simulink model "bmw_roadster"  (R2022b)
settings: Solver=ode45  StartTime=0.0  StopTime=15  RelTol=1e-3  EnableMultiTasking=on
PreLoadFcn:
  | % Parameters
  | load gear_data;
  | FDR = 3.23;
  | AvgEngTorque = 222;
  | Loss = 0.8;
  | r_tire = 1.030;
  | m = 104.2;
  | Cd = 0.4;
  | rho = 2.377e-3;
  | h = 4.15;
  | w = 5.71;
settings Model: Creator=jrivitus  LastModifiedBy=bensweet
settings SolverCC: AlgebraicLoopSolver=TrustRegion
settings DataIOCC: ExternalInput=[t, gear]  LimitDataPoints=on  LoadExternalInput=on  SaveFormat=Array  ReturnWorkspaceOutputs=off
settings OptimizationCC: ExpressionDepthLimit=2147483647  LifeSpan=inf
settings DebuggingCC: UnconnectedInputMsg=warning  UnconnectedOutputMsg=warning  UnconnectedLineMsg=warning  PregeneratedLibrarySubsystemCodeDiagnostic=none  SFMachineParentedDataDiag=warning
settings HardwareCC: ProdBitPerPointer=32  ProdBitPerSizeT=32  ProdBitPerPtrDiffT=32  ProdLargestAtomicFloat=None  ProdIntDivRoundTo=Undefined  ProdEndianess=Unspecified  ProdWordSize=32  ProdHWDeviceType=32-bit Generic
settings ModelReferenceCC: EnableRefExpFcnMdlSchedulingChecks=on  PropagateSignalLabelsOutOfModel=off
settings SFSimCC: SimUseLocalCustomCode=off
settings RTWCC: RTWUseLocalCustomCode=off  DLArmComputeVersion=19.05
settings CodeAppCC: StateflowObjectComments=on
settings GRTTargetCC: TargetLangStandard=C89/C90 (ANSI)  CombineOutputUpdateFcns=off  GRTInterface=on
settings ConfigComp: CovMetricSettings=dw  CovSaveCumulativeToWorkspaceVar=on  CovSaveSingleToWorkspaceVar=on  CovExternalEMLEnable=off  CovSFcnEnable=off

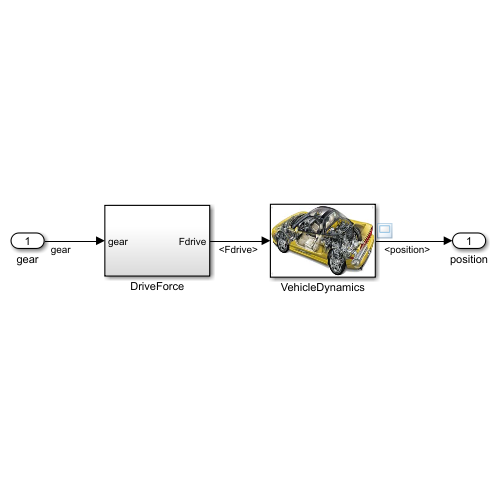
[thumbnail: Simulink's stored preview of the top-level diagram]
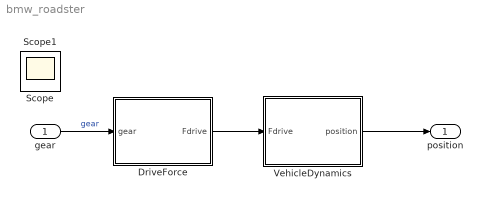
== system bmw_roadster ==
  gear : Inport
  DriveForce : Subsystem
  VehicleDynamics : Subsystem
      mask Display: image("carImg.jpg")
  position : Outport  VectorParamsAs1DForOutWhenUnconnected=off
  Scope : Scope
  Scope1 : Scope
  wires:
  DriveForce/1(Fdrive) -> VehicleDynamics/1(Fdrive)
  gear/1 -> DriveForce/1(gear)  "gear"
  VehicleDynamics/1(position) -> position/1

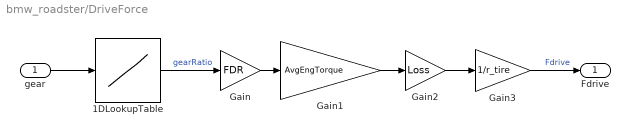
== system bmw_roadster/DriveForce ==
  gear : Inport
  1DLookupTable : Lookup_n-D  NumberOfTableDimensions=1  BreakpointsForDimension1=[1:5]  Table=[4.21 2.49 1.66 1.24 1.00]  InterpMethod=Flat  ExtrapMethod=Clip  RndMeth=Simplest
  Gain : Gain  Gain=FDR
  Gain1 : Gain  Gain=AvgEngTorque
  Gain2 : Gain  Gain=Loss
  Gain3 : Gain  Gain=1/r_tire
  Fdrive : Outport  VectorParamsAs1DForOutWhenUnconnected=off
  wires:
  gear/1 -> 1DLookupTable/1
  1DLookupTable/1 -> Gain/1  "gearRatio"
  Gain/1 -> Gain1/1
  Gain1/1 -> Gain2/1
  Gain2/1 -> Gain3/1
  Gain3/1 -> Fdrive/1  "Fdrive"

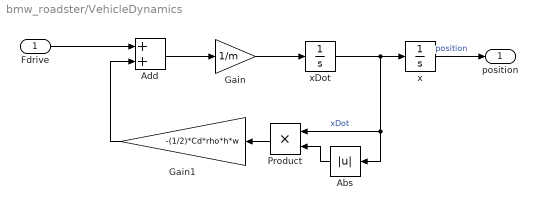
== system bmw_roadster/VehicleDynamics ==
  Fdrive : Inport
  Abs : Abs  SaturateOnIntegerOverflow=off
  Add : Sum
  Gain : Gain  Gain=1/m
  Gain1 : Gain  Gain=-(1/2)*Cd*rho*h*w
  Product : Product  RndMeth=Zero
  x : Integrator
  xDot : Integrator
  position : Outport  VectorParamsAs1DForOutWhenUnconnected=off
  wires:
  xDot/1 -> x/1, Product/1, Abs/1  "xDot"
  x/1 -> position/1  "position"
  Add/1 -> Gain/1
  Gain/1 -> xDot/1
  Abs/1 -> Product/2
  Product/1 -> Gain1/1
  Gain1/1 -> Add/2
  Fdrive/1 -> Add/1
